simulink model "zad1"  (R2024b)
settings: Solver=VariableStepAuto  StartTime=0.0  StopTime=30  MaxStep=0.01  RelTol=1e-3
values from neighbouring files (symbols this model uses):
  Kp = 0.6*Kkr    (= 10.92)    [dane.m]    (also in lab2.m = 6)
  Td = 0.125*Tosc    (= 0.39125)    [dane.m]    (also in lab2.m = 2.475)
  Ti = 0.5*Tosc    (= 1.565)    [dane.m]    (also in lab2.m = 1.1)
settings Model: Creator=marci  LastModifiedBy=marci

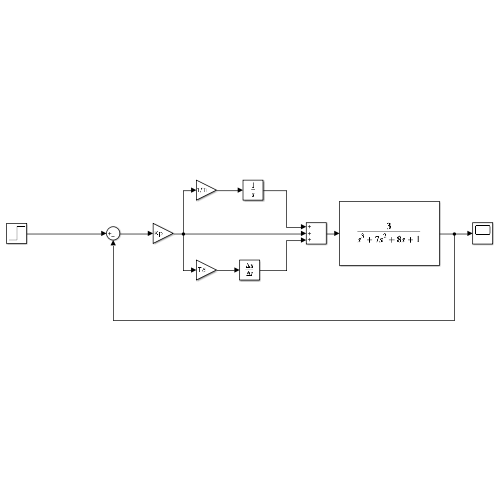
[thumbnail: Simulink's stored preview of the top-level diagram]
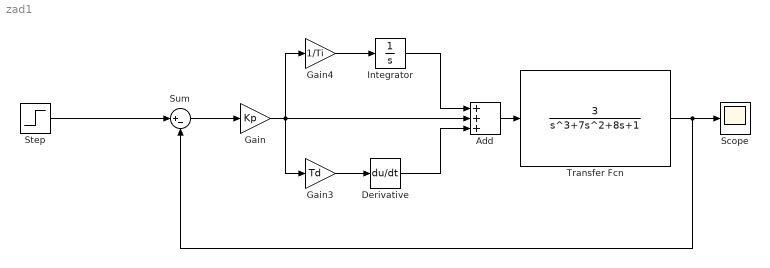
== system zad1 ==
  Add : Sum  Inputs=+++
  Derivative : Derivative
  Gain : Gain  Gain=Kp
  Gain3 : Gain  Gain=Td
  Gain4 : Gain  Gain=1/Ti
  Integrator : Integrator
  Scope : Scope
  Step : Step  SampleTime=0
  Sum : Sum  Inputs=|+-
  Transfer Fcn : TransferFcn  Numerator=[3]  Denominator=[1 7 8 1]
  wires:
  Step/1 -> Sum/1
  Sum/1 -> Gain/1
  Gain/1 -> Add/2, Gain4/1, Gain3/1
  Gain3/1 -> Derivative/1
  Gain4/1 -> Integrator/1
  Integrator/1 -> Add/1
  Derivative/1 -> Add/3
  Add/1 -> Transfer Fcn/1
  Transfer Fcn/1 -> Sum/2, Scope/1
